simulink model "cruise_model"  (R2017a)
settings: Solver=VariableStepAuto  StartTime=0.0  StopTime=40  RelTol=1e-3
model workspace: external: MAT-File /home/nikhil/breach_master/Examples/Cruise-control-design-using-PID-master/cc_expanded.mat (data not in the file)
undefined symbols (not defined in the file or in its folder): D, DOutMax, DOutMin, I, InitialConditionForFilter, InitialConditionForIntegrator, IOutMax, IOutMin, N, NOutMax, NOutMin, P, POutMax, POutMin, SampleTime, SumDOutMax, SumDOutMin, SumOutMax, SumOutMin
libraries: simulink x1
settings Model: Creator=root  LastModifiedBy=nikhil

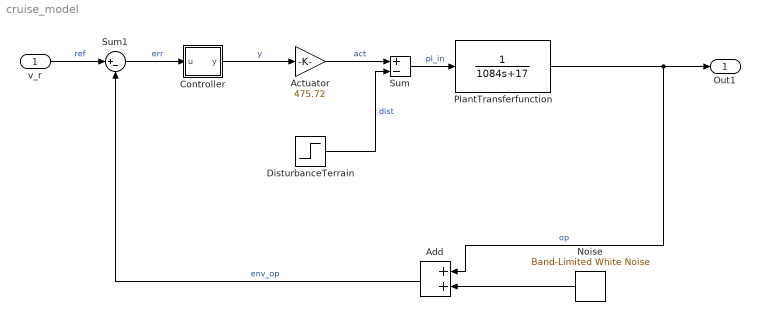
== system cruise_model ==
  v_r : Inport
  " Noise" : simulink/Sources/Band-Limited White Noise  Cov=[0.01]  Ts=0.1  seed=[23341]
  Actuator : Gain  Gain=475.72
  Add : Sum
  Controller : Subsystem
  DisturbanceTerrain : Step  Time=350  After=475.72*9.81*sin(pi/45)  SampleTime=0
  PlantTransferfunction : TransferFcn  Denominator=[1084 17]
  Sum : Sum  Inputs=+-
  Sum1 : Sum  Inputs=|+-
  Out1 : Outport
  wires:
  Actuator/1 -> Sum/1  "act"
  PlantTransferfunction/1 -> Out1/1, Add/1  "op"
  DisturbanceTerrain/1 -> Sum/2  "dist"
  Sum/1 -> PlantTransferfunction/1  "pl_in"
  Controller/1(y) -> Actuator/1  "y"
  " Noise"/1 -> Add/2
  Add/1 -> Sum1/2  "env_op"
  Sum1/1 -> Controller/1(u)  "err"
  v_r/1 -> Sum1/1  "ref"

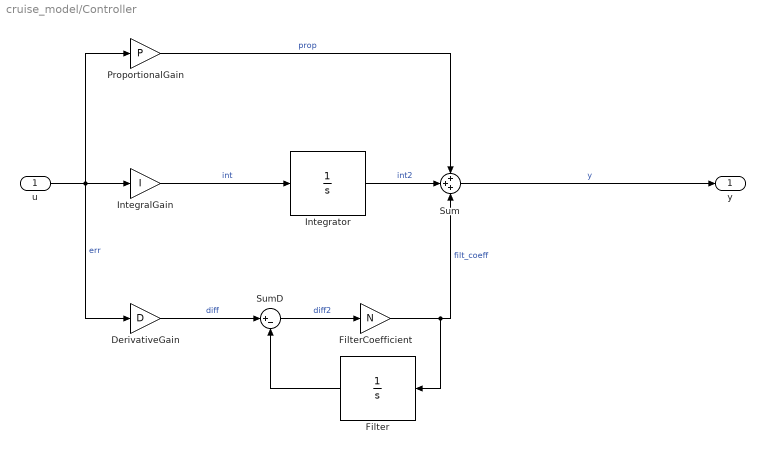
== system cruise_model/Controller ==
  u : Inport
  DerivativeGain : Gain  DisableCoverage=on  Gain=D  ParamMin=DParamMin  ParamMax=DParamMax  OutMin=DOutMin  OutMax=DOutMax
  Filter : Integrator  DisableCoverage=on  InitialCondition=InitialConditionForFilter
  FilterCoefficient : Gain  Gain=N  ParamMin=NParamMin  ParamMax=NParamMax  OutMin=NOutMin  OutMax=NOutMax  SampleTime=SampleTime
  IntegralGain : Gain  DisableCoverage=on  Gain=I  ParamMin=IParamMin  ParamMax=IParamMax  OutMin=IOutMin  OutMax=IOutMax  SampleTime=SampleTime
  Integrator : Integrator  InitialCondition=InitialConditionForIntegrator
  ProportionalGain : Gain  Gain=P  ParamMin=PParamMin  ParamMax=PParamMax  OutMin=POutMin  OutMax=POutMax  SampleTime=SampleTime
  Sum : Sum  Inputs=+++  OutMin=SumOutMin  OutMax=SumOutMax  SampleTime=SampleTime
  SumD : Sum  DisableCoverage=on  Inputs=|+-  OutMin=SumDOutMin  OutMax=SumDOutMax  SampleTime=SampleTime
  y : Outport  SampleTime=SampleTime  InitialOutput=0
  wires:
  Sum/1 -> y/1  "y"
  Integrator/1 -> Sum/2  "int2"
  ProportionalGain/1 -> Sum/1  "prop"
  SumD/1 -> FilterCoefficient/1  "diff2"
  IntegralGain/1 -> Integrator/1  "int"
  FilterCoefficient/1 -> Sum/3, Filter/1  "filt_coeff"
  Filter/1 -> SumD/2
  DerivativeGain/1 -> SumD/1  "diff"
  u/1 -> ProportionalGain/1, DerivativeGain/1, IntegralGain/1  "err"
